simulink model "sim_ex5"  (R2015b)
settings: Solver=ode23t  StartTime=0.0  StopTime=0.5  RelTol=1e-3
values from neighbouring files (symbols this model uses):
  df = 0.0001    [ex1.m]    (also in ex5.m)
  J1 = 1.8e-5    (= 1.8e-05)    [ex1.m]    (also in ex5.m)
  J2 = 1.8e-5    (= 1.8e-05)    [ex1.m]    (also in ex5.m)
  kf = 0.05    [ex1.m]    (also in ex5.m)
  motor_L = motor_pars    [ex1.m]
  n = 5    [ex1.m]    (also in ex5.m)
  sim_V = 24    [ex1.m]    (also in ex5.m)
settings Model: Creator=gabras  LastModifiedBy=Lamn
settings DataIOCC: SaveFormat=Array
settings DebuggingCC: SolverPrmCheckMsg=warning
settings HardwareCC: ProdBitPerPointer=32  ProdLargestAtomicFloat=None  ProdIntDivRoundTo=Undefined  ProdEndianess=Unspecified  ProdWordSize=32  ProdHWDeviceType=32-bit Generic
settings GRTTargetCC: GeneratePreprocessorConditionals=Disable all
settings ConfigComp: CovModelRefEnable=Off  CovSFcnEnable=off

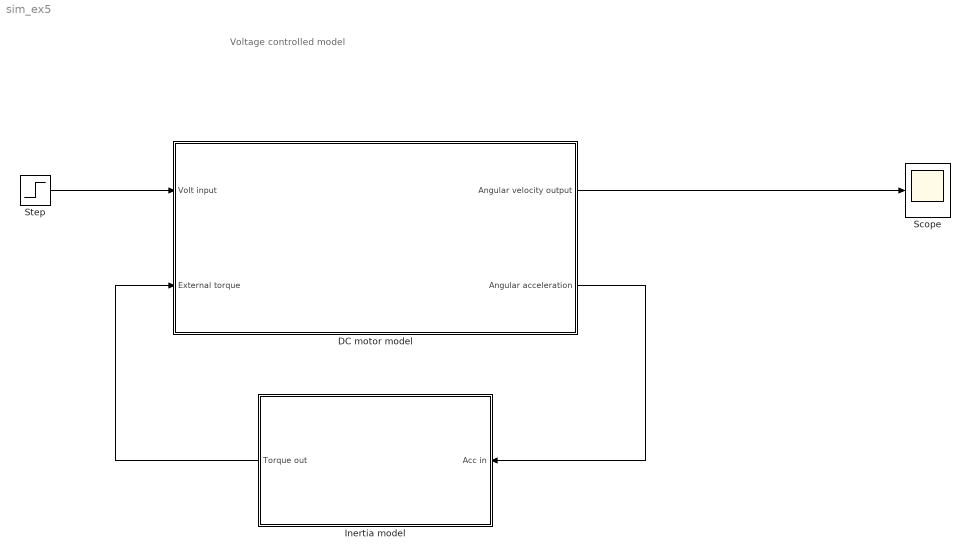
== system sim_ex5 ==
  note: Voltage controlled model
  DC motor model : Subsystem
  Inertia model : Subsystem
  Scope : Scope
  Step : Step  Time=0  After=sim_V  SampleTime=0
  wires:
  Step/1 -> DC motor model/1("Volt input ")
  DC motor model/1("Angular velocity output ") -> Scope/1
  Inertia model/1(Torque out) -> DC motor model/2(External torque)
  DC motor model/2("Angular acceleration ") -> Inertia model/1(Acc in)

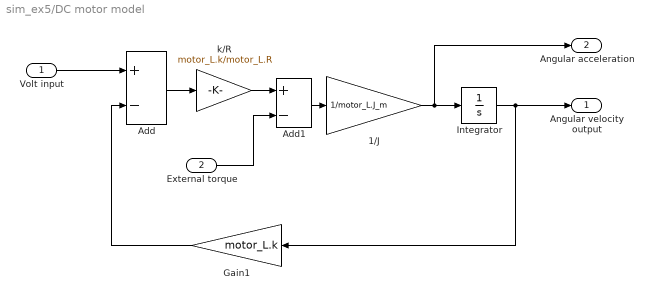
== system sim_ex5/DC motor model ==
  "Volt input " : Inport
  External torque : Inport  Port=2
  1/J : Gain  Gain=1/motor_L.J_m
  Add : Sum  Inputs=+-
  Add1 : Sum  Inputs=+-
  Gain1 : Gain  Gain=motor_L.k
  Integrator : Integrator
  "k/R " : Gain  Gain=motor_L.k/motor_L.R
  "Angular velocity output " : Outport
  "Angular acceleration " : Outport  Port=2
  wires:
  "Volt input "/1 -> Add/1
  Gain1/1 -> Add/2
  Add/1 -> "k/R "/1
  "k/R "/1 -> Add1/1
  Add1/1 -> 1/J/1
  1/J/1 -> Integrator/1, "Angular acceleration "/1
  Integrator/1 -> Gain1/1, "Angular velocity output "/1
  External torque/1 -> Add1/2

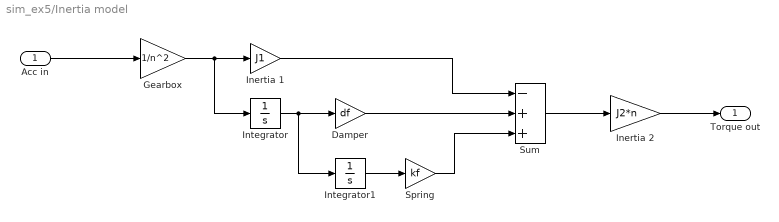
== system sim_ex5/Inertia model ==
  Acc in : Inport
  Damper : Gain  Gain=df
  Gearbox : Gain  Gain=1/n^2
  Inertia 1 : Gain  Gain=J1
  Inertia 2 : Gain  Gain=J2*n
  Integrator : Integrator
  Integrator1 : Integrator
  Spring : Gain  Gain=kf
  Sum : Sum  Inputs=-++
  Torque out : Outport
  wires:
  Acc in/1 -> Gearbox/1
  Inertia 1/1 -> Sum/1
  Integrator1/1 -> Spring/1
  Spring/1 -> Sum/3
  Damper/1 -> Sum/2
  Integrator/1 -> Damper/1, Integrator1/1
  Gearbox/1 -> Integrator/1, Inertia 1/1
  Sum/1 -> Inertia 2/1
  Inertia 2/1 -> Torque out/1
